simulink model "mass_spring_damper_MPC"  (R2019b)
settings: Solver=VariableStepAuto  StartTime=0.0  StopTime=10  RelTol=1e-3
libraries: mpclib x1
settings Model: Creator=Murray  LastModifiedBy=Murray

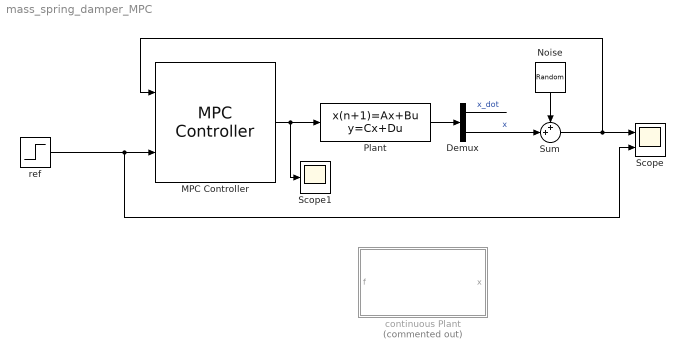
== system mass_spring_damper_MPC ==
  Demux : Demux  Outputs=2
  MPC Controller : mpclib/MPC Controller  SCDEnableBlockLinearizationSpecification=on  mpcobj=mpc1  is_multiple=0  enable_value=0  return_u0=off  updateMPCinCallerWorkspace=on  md_inport=off  mv_inport=off  uref_inport=off  return_cost=off  return_mvseq=off  return_qpstatus=off  return_xseq=off  return_state=off  return_ovseq=off  state_inport=off  umin_inport=off  umax_inport=off  ymin_inport=off  ymax_inport=off  cc_inport=off  ywt_inport=off  uwt_inport=off  duwt_inport=off  rhoeps_inport=off  pm_inport=off  MaximumP=20  HorizonChoice=FixedHorizon  n_ts=0.1  n_p=20  n_mv=1  n_md=0  n_ud=0  n_mo=1  n_uo=0  BlockDataType=double  SampleTimeInherited=off  switch_inport=off
  Noise : RandomNumber  Variance=0.00001  SampleTime=0.01
  Plant : DiscreteStateSpace  A="[0.9271  -0.4837;  0.09673  0.9755]"  B="[0.09673;  0.004897]"  C="[1  0;  0 1]"  D=[0; 0]  SampleTime=0.1
  Scope : Scope  NumInputPorts=2
  Scope1 : Scope
  Sum : Sum  Inputs=++|
  continuous Plant : Subsystem  Commented=on
  ref : Step  SampleTime=0
  wires:
  ref/1 -> Scope/2, MPC Controller/2
  MPC Controller/1 -> Plant/1, Scope1/1
  Sum/1 -> MPC Controller/1, Scope/1
  Noise/1 -> Sum/1
  Demux/2 -> Sum/2  "x"
  Plant/1 -> Demux/1
  Demux/1 -> ?  "x_dot"

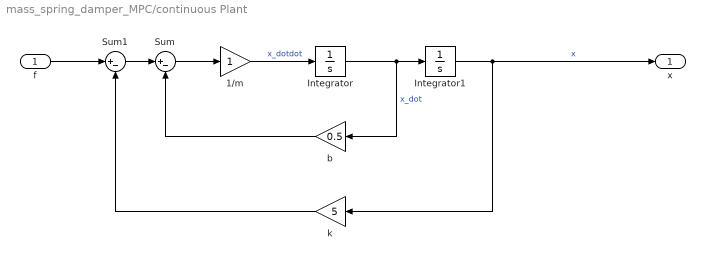
== system mass_spring_damper_MPC/continuous Plant ==
  f : Inport
  1/m : Gain
  Integrator : Integrator
  Integrator1 : Integrator
  Sum : Sum  Inputs=|+-
  Sum1 : Sum  Inputs=|+-
  b : Gain  Gain=0.5
  k : Gain  Gain=5
  x : Outport
  wires:
  f/1 -> Sum1/1
  Integrator/1 -> b/1, Integrator1/1  "x_dot"
  Sum1/1 -> Sum/1
  1/m/1 -> Integrator/1  "x_dotdot"
  Integrator1/1 -> x/1, k/1  "x"
  Sum/1 -> 1/m/1
  b/1 -> Sum/2
  k/1 -> Sum1/2
